simulink model "SpaceVectorPWM"  (R2022a)
settings: Solver=VariableStepAuto  StartTime=0.0  StopTime=0.5  RelTol=1e-5
model workspace (MAT data in the model file):
  Mindex = 0.795982752482
  Modulation = 5
libraries: simulink x13, spsIGBTDiodeLib x6, spsSeriesRLCBranchLib x3, spsDCVoltageSourceLib x2, spsAsynchronousMachineSIUnitsLib x1, spsMeanLib x1, spsRMSLib x1, spsGroundLib x1, spsThreePhaseVIMeasurementLib x1, spsVoltageMeasurementLib x1, spspowerguiLib x1
settings Model: Creator=Alperen  LastModifiedBy=Alperen
settings SolverCC: AlgebraicLoopSolver=TrustRegion
settings DebuggingCC: MaxConsecutiveZCsMsg=none  ModelReferenceExtraNoncontSigs=none
settings RTWCC: DLArmComputeVersion=19.05

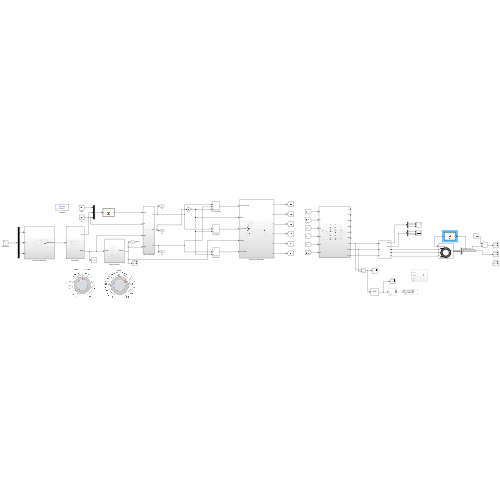
[thumbnail: Simulink's stored preview of the top-level diagram]
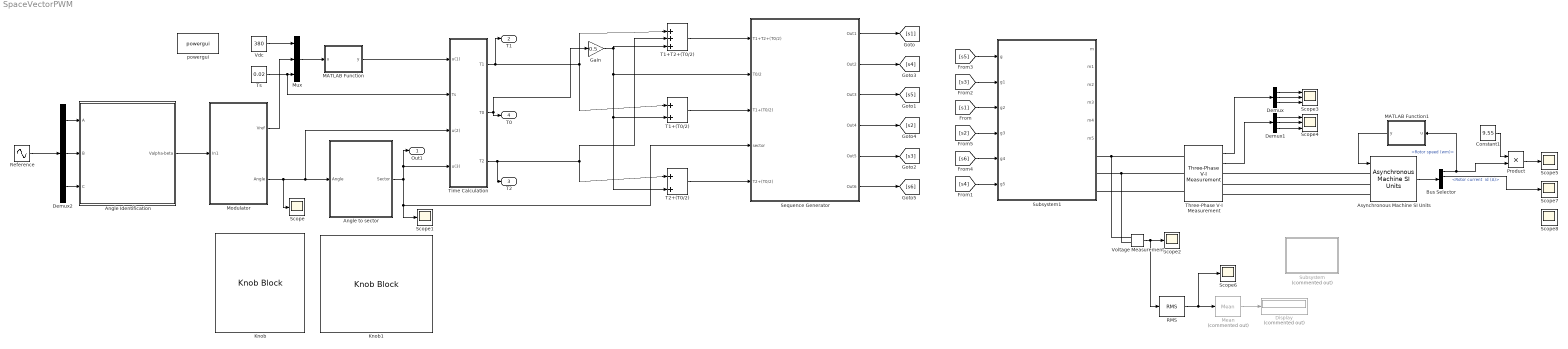
== system SpaceVectorPWM ==
  Angle Identification : Subsystem
  Angle to sector : Subsystem
  Asynchronous Machine SI Units : spsAsynchronousMachineSIUnitsLib/Asynchronous Machine SI Units  RotorType=Squirrel-cage  PresetModel="15:  5.4 HP (4KW)   400 V  50Hz 1430 RPM"  MechanicalLoad=Torque Tm  ShowDetailedParameters=on  ReferenceFrame=Rotor  Units=SI  MeasurementBus=off  NominalParameters=[4000 400 50]  VoltageRatio=1  Stator=[1.405 0.005839]  Rotor=[1.395 0.005839]  Cage1=[0.4155 0.002066]  Cage2=[0.4168 0.0003495]  Lm=0.1722  Mechanical=[0.0131 0.002985 2]  PolePairs=2  InitialConditions=[0 0 0 0 0 0 0 0]  SimulateSaturation=off  Saturation=[14.03593122, 27.81365428, 53.79336849, 72.68890987, 97.98006896, 148.6815601, 215.7428561, 302.9841135, 428.7778367 ; 230, 322, 414, 460, 506, 552, 598, 644, 690]  LoadFlowParameters=1492000  TsPowergui=0  TsBlock=-1  IterativeModel=Trapezoidal non iterative  IterativeDiscreteModel=Trapezoidal non iterative  Pmec=1.492e+006
  Bus Selector : BusSelector  OutputSignals="Mechanical.Rotor speed (wm),Rotor measurements.Rotor current  id (A),Rotor measurements.Rotor current  iq (A),Mechanical.Electromagnetic torque Te (N*m)"
  Constant1 : Constant  Value=9.55
  Demux : Demux  Outputs=3
  Demux1 : Demux  Outputs=3
  Demux2 : Demux  Outputs=3
  Display : Display  Commented=on
  Gain : Gain  Gain=0.5
  Knob : KnobBlock  TickInterval=5
  Knob1 : KnobBlock  ScaleMax=1.15  TickInterval=0.05
  MATLAB Function : MATLAB Function  TreatAsAtomicUnit=on
  MATLAB Function1 : MATLAB Function  TreatAsAtomicUnit=on
  Mean : spsMeanLib/Mean  Commented=on  Freq=50  Vinit=0  Ts=0
  Modulator : Subsystem
  Mux : Mux  Inputs=3
  Product : Product
  RMS : spsRMSLib/RMS  TrueRMS=on  Freq=50  RMSInit=390  Ts=0
  Reference : Sin  Amplitude=230  Frequency=49.62226359049479  Phase=[0 -2*pi/3 -4*pi/3]  SampleTime=0
  Scope{,1..2,5..8} (7 alike) : Scope
  Scope3 : Scope  NumInputPorts=3
  Scope4 : Scope  NumInputPorts=3
  Sequence Generator : Subsystem
  Subsystem : Subsystem  Commented=on
  Subsystem1 : Subsystem
  T1+(T0/2) : Sum  Inputs=|++
  T1+T2+(T0/2) : Sum  Inputs=|+++
  T2+(T0/2) : Sum  Inputs=|++
  Three-Phase V-I Measurement : spsThreePhaseVIMeasurementLib/Three-Phase V-I Measurement  VoltageMeasurement=phase-to-phase  SetLabelV=off  LabelV=Vabc  Vpu=off  VpuLL=off  CurrentMeasurement=yes  SetLabelI=off  LabelI=Iabc  Ipu=off  Pbase=100e6  Vbase=500e3  OutputType=Complex  PhasorSimulation=off  PSBequivalent=0
  Time Calculation : Subsystem
  Ts : Constant  Value=0.02
  Vdc : Constant  Value=380
  Voltage Measurement : spsVoltageMeasurementLib/Voltage Measurement  PhasorSimulation=off  OutputType=Complex  PSBequivalent=0
  powergui : spspowerguiLib/powergui  Priority=1  SimulationMode=Discrete  SampleTime=1e-6  frequency=60  Iterations=50  frequencyindice=0  Pbase=100e6  ErrMax=1e-4  UnitsV=kV  UnitsW=MW  buscounter=0  FunctionMessages=off  echomessages=off  EnableUseOfTLC=off  CurrentSourceSwitches=off  DisableSnubberDevices=off  DisableRonSwitches=off  DisableVfSwitches=off  DisplayEquations=off  AutomaticDiscreteSolvers=off  SolverType=Tustin/Backward Euler (TBE)  Interpol=off  ExternalGateDelay=off  methode=off  Ts=100  x0status=blocks  SPID=on  SwTol=0  HookPort=off  NonlinearTolerance=1e-4  nMaxIteration=100  ContinueOnMaxIteration=off  RestoreLinks=warning  ResistiveCurrentMeasurement=off  Frange=[0:2:500]  Ylog=off  Xlog=on  ShowGrid=off  save=off  variable=ZData  structure=0  ZoomFFT=off  StartTime=0.0  cycles=1  DisplayStyle=1  fundamental=60  FreqAxis=off  MaxFrequency=1000  frequencyindicesteady=1  RmsSteady=1  display=off
  Out1 : Outport  SignalName=sector
  T1 : Outport  Port=2
  T2 : Outport  Port=3
  T0 : Outport  Port=4
  wires:
  Angle Identification/1(Valpha-beta) -> Modulator/1(In1)
  Modulator/1(Vref) -> Mux/2
  Modulator/2(Angle) -> Time Calculation/3(u(2)), Angle to sector/1(Angle), Scope/1
  Angle to sector/1(Sector) -> Out1/1, Time Calculation/4(u(3)), Sequence Generator/4(sector), Scope1/1
  Vdc/1 -> Mux/1
  Ts/1 -> Time Calculation/2(Ts), Mux/3
  Mux/1 -> MATLAB Function/1(u)
  MATLAB Function/1(y) -> Time Calculation/1(u(1))
  Time Calculation/1(T1) -> T1/1, T1+(T0/2)/1, T1+T2+(T0/2)/1
  Time Calculation/2(T0) -> Gain/1, T0/1
  Time Calculation/3(T2) -> T2/1, T1+T2+(T0/2)/2, T2+(T0/2)/1
  Gain/1 -> T1+T2+(T0/2)/3, T1+(T0/2)/2, T2+(T0/2)/2, Sequence Generator/2(T0/2)
  Three-Phase V-I Measurement/2 -> Demux1/1
  Demux1/3 -> Scope4/3
  Demux1/1 -> Scope4/1
  Demux1/2 -> Scope4/2
  [s3] -> Subsystem1/2(g1)
  Demux/1 -> Scope3/1
  [s5] -> Subsystem1/1(g)
  Demux/2 -> Scope3/2
  [s6] -> Subsystem1/5(g4)
  [s2] -> Subsystem1/4(g3)
  [s1] -> Subsystem1/3(g2)
  [s4] -> Subsystem1/6(g5)
  Demux/3 -> Scope3/3
  T1+T2+(T0/2)/1 -> Sequence Generator/1(T1+T2+(T0/2))
  T1+(T0/2)/1 -> Sequence Generator/3(T1+(T0/2))
  T2+(T0/2)/1 -> Sequence Generator/5(T2+(T0/2))
  Sequence Generator/1(Out1) -> [s1]
  Sequence Generator/2(Out2) -> [s4]
  Sequence Generator/3(Out3) -> [s5]
  Sequence Generator/4(Out4) -> [s2]
  Sequence Generator/5(Out5) -> [s3]
  Sequence Generator/6(Out6) -> [s6]
  Reference/1 -> Demux2/1
  Demux2/3 -> Angle Identification/3(C)
  Demux2/2 -> Angle Identification/2(B)
  Demux2/1 -> Angle Identification/1(A)
  RMS/1 -> Scope6/1, Mean/1
  Voltage Measurement/1 -> RMS/1, Scope2/1
  Mean/1 -> Display/1
  Three-Phase V-I Measurement/1 -> Demux/1
  Asynchronous Machine SI Units/1 -> Bus Selector/1
  Constant1/1 -> Product/1
  Bus Selector/1 -> MATLAB Function1/1(u), Product/2  "<Rotor speed (wm)>"
  Bus Selector/2 -> Scope7/1  "<Rotor current  id (A)>"
  Product/1 -> Scope5/1
  MATLAB Function1/1(y) -> Asynchronous Machine SI Units/1
  connections:
  Three-Phase V-I Measurement/LConn3 -- Subsystem1/RConn3
  Three-Phase V-I Measurement/LConn2 -- Voltage Measurement/LConn2 -- Subsystem1/RConn2
  Three-Phase V-I Measurement/LConn1 -- Voltage Measurement/LConn1 -- Subsystem1/RConn1
  Asynchronous Machine SI Units/LConn3 -- Three-Phase V-I Measurement/RConn3
  Asynchronous Machine SI Units/LConn2 -- Three-Phase V-I Measurement/RConn2
  Asynchronous Machine SI Units/LConn1 -- Three-Phase V-I Measurement/RConn1

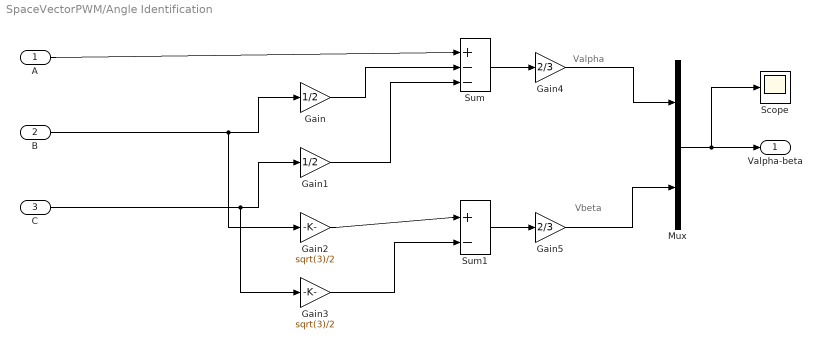
== system SpaceVectorPWM/Angle Identification ==
  note: Valpha
  note: Vbeta
  A : Inport
  B : Inport  Port=2
  C : Inport  Port=3
  Gain : Gain  Gain=1/2
  Gain1 : Gain  Gain=1/2
  Gain2 : Gain  Gain=sqrt(3)/2
  Gain3 : Gain  Gain=sqrt(3)/2
  Gain4 : Gain  Gain=2/3
  Gain5 : Gain  Gain=2/3
  Mux : Mux  Inputs=2
  Scope : Scope
  Sum : Sum  Inputs=|+--
  Sum1 : Sum  Inputs=|+-
  Valpha-beta : Outport
  wires:
  A/1 -> Sum/1
  C/1 -> Gain3/1, Gain1/1
  Sum/1 -> Gain4/1
  Gain/1 -> Sum/2
  Gain1/1 -> Sum/3
  B/1 -> Gain2/1, Gain/1
  Gain4/1 -> Mux/1
  Gain2/1 -> Sum1/1
  Gain3/1 -> Sum1/2
  Sum1/1 -> Gain5/1
  Gain5/1 -> Mux/2
  Mux/1 -> Scope/1, Valpha-beta/1

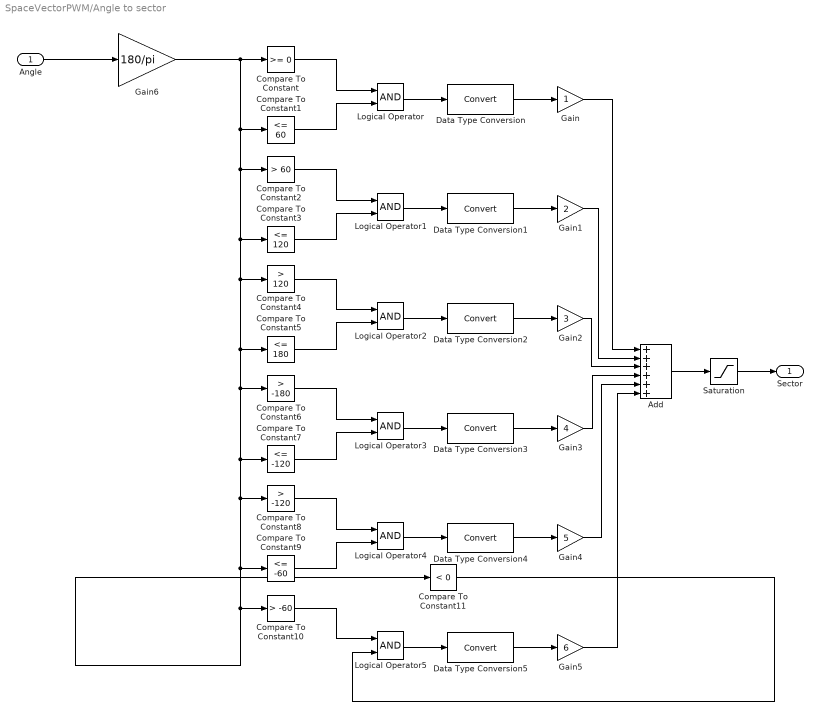
== system SpaceVectorPWM/Angle to sector ==
  Angle : Inport
  Add : Sum  Inputs=++++++
  Compare To Constant : simulink/Logic and Bit Operations/Compare To Constant  relop=>=  const=0  OutDataTypeStr=boolean
  Compare To Constant1 : simulink/Logic and Bit Operations/Compare To Constant  relop=<=  const=60  OutDataTypeStr=boolean
  Compare To Constant10 : simulink/Logic and Bit Operations/Compare To Constant  relop=>  const=-60  OutDataTypeStr=boolean
  Compare To Constant11 : simulink/Logic and Bit Operations/Compare To Constant  relop=<  const=0  OutDataTypeStr=boolean
  Compare To Constant2 : simulink/Logic and Bit Operations/Compare To Constant  relop=>  const=60  OutDataTypeStr=boolean
  Compare To Constant3 : simulink/Logic and Bit Operations/Compare To Constant  relop=<=  const=120  OutDataTypeStr=boolean
  Compare To Constant4 : simulink/Logic and Bit Operations/Compare To Constant  relop=>  const=120  OutDataTypeStr=boolean
  Compare To Constant5 : simulink/Logic and Bit Operations/Compare To Constant  relop=<=  const=180  OutDataTypeStr=boolean
  Compare To Constant6 : simulink/Logic and Bit Operations/Compare To Constant  relop=>  const=-180  OutDataTypeStr=boolean
  Compare To Constant7 : simulink/Logic and Bit Operations/Compare To Constant  relop=<=  const=-120  OutDataTypeStr=boolean
  Compare To Constant8 : simulink/Logic and Bit Operations/Compare To Constant  relop=>  const=-120  OutDataTypeStr=boolean
  Compare To Constant9 : simulink/Logic and Bit Operations/Compare To Constant  relop=<=  const=-60  OutDataTypeStr=boolean
  Data Type Conversion{,1..5} (6 alike) : DataTypeConversion  SaturateOnIntegerOverflow=off  RndMeth=Floor
  Gain : Gain
  Gain1 : Gain  Gain=2
  Gain2 : Gain  Gain=3
  Gain3 : Gain  Gain=4
  Gain4 : Gain  Gain=5
  Gain5 : Gain  Gain=6
  Gain6 : Gain  Gain=180/pi
  Logical Operator{,1..5} (6 alike) : Logic  AllPortsSameDT=off  OutDataTypeStr=boolean
  Saturation : Saturate  UpperLimit=6  LowerLimit=1
  Sector : Outport
  wires:
  Compare To Constant9/1 -> Logical Operator4/2
  Compare To Constant11/1 -> Logical Operator5/2
  Logical Operator5/1 -> Data Type Conversion5/1
  Compare To Constant2/1 -> Logical Operator1/1
  Angle/1 -> Gain6/1
  Compare To Constant3/1 -> Logical Operator1/2
  Gain6/1 -> Compare To Constant11/1, Compare To Constant10/1, Compare To Constant9/1, Compare To Constant8/1, Compare To Constant7/1, Compare To Constant6/1, Compare To Constant5/1, Compare To Constant4/1, Compare To Constant3/1, Compare To Constant2/1, Compare To Constant1/1, Compare To Constant/1
  Compare To Constant1/1 -> Logical Operator/2
  Gain3/1 -> Add/4
  Logical Operator/1 -> Data Type Conversion/1
  Data Type Conversion1/1 -> Gain1/1
  Logical Operator2/1 -> Data Type Conversion2/1
  Data Type Conversion2/1 -> Gain2/1
  Logical Operator4/1 -> Data Type Conversion4/1
  Compare To Constant5/1 -> Logical Operator2/2
  Data Type Conversion/1 -> Gain/1
  Compare To Constant8/1 -> Logical Operator4/1
  Data Type Conversion4/1 -> Gain4/1
  Logical Operator3/1 -> Data Type Conversion3/1
  Gain/1 -> Add/1
  Logical Operator1/1 -> Data Type Conversion1/1
  Compare To Constant6/1 -> Logical Operator3/1
  Data Type Conversion5/1 -> Gain5/1
  Compare To Constant/1 -> Logical Operator/1
  Data Type Conversion3/1 -> Gain3/1
  Compare To Constant7/1 -> Logical Operator3/2
  Gain2/1 -> Add/3
  Compare To Constant4/1 -> Logical Operator2/1
  Gain1/1 -> Add/2
  Compare To Constant10/1 -> Logical Operator5/1
  Gain4/1 -> Add/5
  Gain5/1 -> Add/6
  Add/1 -> Saturation/1
  Saturation/1 -> Sector/1

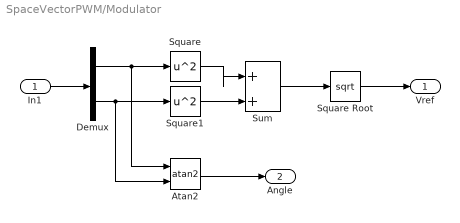
== system SpaceVectorPWM/Modulator ==
  In1 : Inport
  Atan2 : Trigonometry  Operator=atan2
  Demux : Demux  Outputs=2
  Square : Math  Operator=square
  Square Root : Sqrt
  Square1 : Math  Operator=square
  Sum : Sum  Inputs=|++
  Vref : Outport
  Angle : Outport  Port=2
  wires:
  Square Root/1 -> Vref/1
  Demux/1 -> Atan2/1, Square/1
  Demux/2 -> Atan2/2, Square1/1
  Square/1 -> Sum/1
  Sum/1 -> Square Root/1
  Square1/1 -> Sum/2
  Atan2/1 -> Angle/1
  In1/1 -> Demux/1

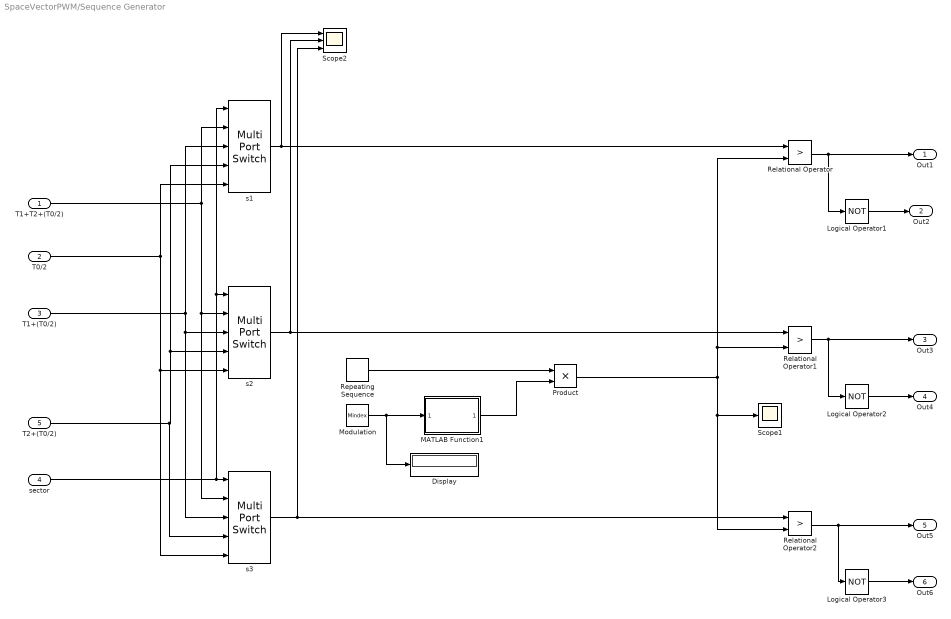
== system SpaceVectorPWM/Sequence Generator ==
  T1+T2+(T0/2) : Inport
  T0/2 : Inport  Port=2
  T1+(T0/2) : Inport  Port=3
  sector : Inport  Port=4
  T2+(T0/2) : Inport  Port=5
  Display : Display
  Logical Operator1 : Logic  Operator=NOT  AllPortsSameDT=off  OutDataTypeStr=boolean
  Logical Operator2 : Logic  Operator=NOT  AllPortsSameDT=off  OutDataTypeStr=boolean
  Logical Operator3 : Logic  Operator=NOT  AllPortsSameDT=off  OutDataTypeStr=boolean
  MATLAB Function1 : MATLAB Function  TreatAsAtomicUnit=on
  Modulation : Constant  Value=Mindex
  Product : Product
  Relational Operator : RelationalOperator  Operator=>  OutDataTypeStr=boolean  RndMeth=Simplest  InputSameDT=off
  Relational Operator1 : RelationalOperator  Operator=>  OutDataTypeStr=boolean  RndMeth=Simplest  InputSameDT=off
  Relational Operator2 : RelationalOperator  Operator=>  OutDataTypeStr=boolean  RndMeth=Simplest  InputSameDT=off
  Repeating Sequence : simulink/Sources/Repeating Sequence  rep_seq_t=[0 1e-3/4 1e-3/2 (1e-3)*3/4 1e-3]  rep_seq_y=[0,1,0,-1,0]
  Scope1 : Scope
  Scope2 : Scope  NumInputPorts=3
  s1 : MultiPortSwitch  DataPortOrder=Specify indices  Inputs=4  DataPortIndices={[1,6],2,5,[3,4]}  SaturateOnIntegerOverflow=off  InputSameDT=off
  s2 : MultiPortSwitch  DataPortOrder=Specify indices  Inputs=4  DataPortIndices={[2,3],4,1,[5,6]}  SaturateOnIntegerOverflow=off  InputSameDT=off
  s3 : MultiPortSwitch  DataPortOrder=Specify indices  Inputs=4  DataPortIndices={[4,5],6,3,[1,2]}  SaturateOnIntegerOverflow=off  InputSameDT=off
  Out1 : Outport
  Out2 : Outport  Port=2
  Out3 : Outport  Port=3
  Out4 : Outport  Port=4
  Out5 : Outport  Port=5
  Out6 : Outport  Port=6
  wires:
  T0/2/1 -> s1/5, s3/5, s2/5
  s3/1 -> Scope2/3, Relational Operator2/1
  Relational Operator1/1 -> Out3/1, Logical Operator2/1
  T1+(T0/2)/1 -> s3/3, s2/3, s1/3
  s1/1 -> Scope2/1, Relational Operator/1
  sector/1 -> s1/1, s2/1, s3/1
  s2/1 -> Scope2/2, Relational Operator1/1
  T1+T2+(T0/2)/1 -> s1/2, s3/2, s2/2
  Relational Operator/1 -> Out1/1, Logical Operator1/1
  Logical Operator3/1 -> Out6/1
  T2+(T0/2)/1 -> s3/4, s2/4, s1/4
  Relational Operator2/1 -> Out5/1, Logical Operator3/1
  Logical Operator1/1 -> Out2/1
  Logical Operator2/1 -> Out4/1
  Product/1 -> Relational Operator/2, Relational Operator1/2, Scope1/1, Relational Operator2/2
  Repeating Sequence/1 -> Product/1
  Modulation/1 -> Display/1, MATLAB Function1/1(Mindex)
  MATLAB Function1/1(Modulation) -> Product/2

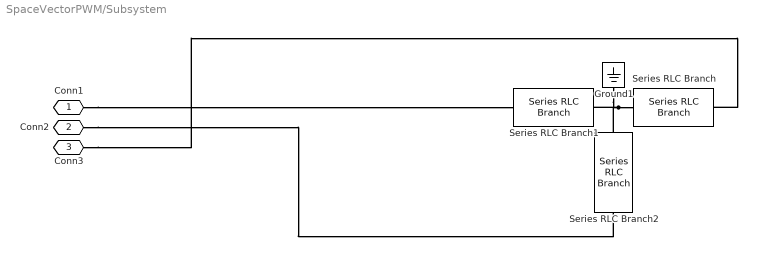
== system SpaceVectorPWM/Subsystem ==
  Ground1 : spsGroundLib/Ground  LConnTagsString=a
  Series RLC Branch : spsSeriesRLCBranchLib/Series RLC Branch  LConnTagsString=__new0  RConnTagsString=__new0  BranchType=RL  Resistance=0.3  Inductance=1e-3  SetiL0=off  InitialCurrent=0  Capacitance=0  Setx0=off  InitialVoltage=0  Measurements=None
  Series RLC Branch1 : spsSeriesRLCBranchLib/Series RLC Branch  LConnTagsString=__new0  RConnTagsString=__new0  BranchType=RL  Resistance=0.3  Inductance=1e-3  SetiL0=off  InitialCurrent=0  Capacitance=0  Setx0=off  InitialVoltage=0  Measurements=None
  Series RLC Branch2 : spsSeriesRLCBranchLib/Series RLC Branch  LConnTagsString=__new0  RConnTagsString=__new0  BranchType=RL  Resistance=0.3  Inductance=1e-3  SetiL0=off  InitialCurrent=0  Capacitance=0  Setx0=off  InitialVoltage=0  Measurements=None
  Conn1 : PMIOPort  Side=Left
  Conn2 : PMIOPort  Port=2  Side=Left
  Conn3 : PMIOPort  Port=3  Side=Left
  connections:
  Series RLC Branch/RConn1 -- Series RLC Branch2/RConn1 -- Series RLC Branch1/RConn1 -- Ground1/LConn1
  Conn3/RConn1 -- Series RLC Branch/LConn1
  Conn1/RConn1 -- Series RLC Branch1/LConn1
  Conn2/RConn1 -- Series RLC Branch2/LConn1

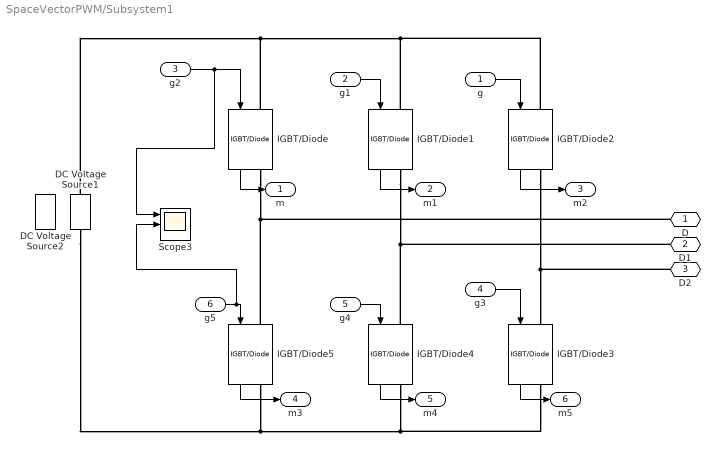
== system SpaceVectorPWM/Subsystem1 ==
  g : Inport
  g1 : Inport  Port=2
  g2 : Inport  Port=3
  g3 : Inport  Port=4
  g4 : Inport  Port=5
  g5 : Inport  Port=6
  DC Voltage Source1 : spsDCVoltageSourceLib/DC Voltage Source  Amplitude=850  Measurements=Voltage
  DC Voltage Source2 : spsDCVoltageSourceLib/DC Voltage Source  Amplitude=400  Measurements=None
  IGBT/Diode{,1..5} (6 alike) : spsIGBTDiodeLib/IGBT//Diode  Ron=1e-5  Rs=1e7  Cs=inf  Measurements=on
  Scope3 : Scope  NumInputPorts=3
  D : PMIOPort  Side=Right
  D1 : PMIOPort  Port=2  Side=Right
  D2 : PMIOPort  Port=3  Side=Right
  m : Outport
  m1 : Outport  Port=2
  m2 : Outport  Port=3
  m3 : Outport  Port=4
  m4 : Outport  Port=5
  m5 : Outport  Port=6
  wires:
  IGBT/Diode5/1 -> m3/1
  IGBT/Diode2/1 -> m2/1
  g2/1 -> Scope3/1, IGBT/Diode/1
  g1/1 -> IGBT/Diode1/1
  g/1 -> IGBT/Diode2/1
  g3/1 -> IGBT/Diode3/1
  g4/1 -> IGBT/Diode4/1
  g5/1 -> Scope3/2, IGBT/Diode5/1
  IGBT/Diode/1 -> m/1
  IGBT/Diode3/1 -> m5/1
  IGBT/Diode4/1 -> m4/1
  IGBT/Diode1/1 -> m1/1
  connections:
  IGBT/Diode5/RConn1 -- DC Voltage Source1/LConn1 -- IGBT/Diode4/RConn1 -- IGBT/Diode3/RConn1
  D2/RConn1 -- IGBT/Diode3/LConn1 -- IGBT/Diode2/RConn1
  D1/RConn1 -- IGBT/Diode4/LConn1 -- IGBT/Diode1/RConn1
  D/RConn1 -- IGBT/Diode5/LConn1 -- IGBT/Diode/RConn1
  IGBT/Diode/LConn1 -- DC Voltage Source1/RConn1 -- IGBT/Diode2/LConn1 -- IGBT/Diode1/LConn1

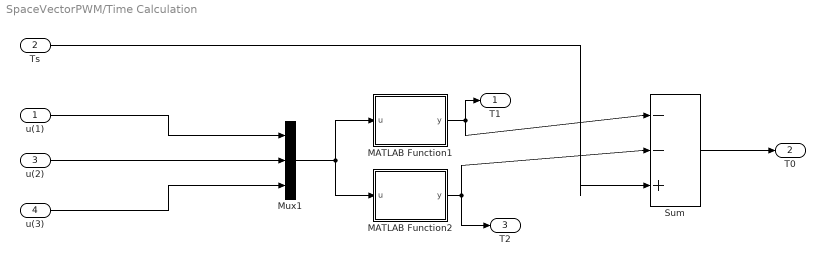
== system SpaceVectorPWM/Time Calculation ==
  u(1) : Inport
  Ts : Inport  Port=2
  u(2) : Inport  Port=3
  u(3) : Inport  Port=4
  MATLAB Function1 : MATLAB Function  TreatAsAtomicUnit=on
  MATLAB Function2 : MATLAB Function  TreatAsAtomicUnit=on
  Mux1 : Mux  Inputs=3
  Sum : Sum  Inputs=|--+
  T1 : Outport
  T0 : Outport  Port=2
  T2 : Outport  Port=3
  wires:
  MATLAB Function2/1(y) -> T2/1, Sum/2
  Sum/1 -> T0/1
  Mux1/1 -> MATLAB Function2/1(u), MATLAB Function1/1(u)
  u(2)/1 -> Mux1/2
  MATLAB Function1/1(y) -> T1/1, Sum/1
  Ts/1 -> Sum/3
  u(3)/1 -> Mux1/3
  u(1)/1 -> Mux1/1

== matlab function SpaceVectorPWM/MATLAB Function ==
  data: u input; y output
function y = fcn(u)
y=sqrt(3)*u(3)*u(2)/u(1);

== matlab function SpaceVectorPWM/Time Calculation/MATLAB Function2 ==
  data: u input; y output
function y = fcn(u)

y=u(1)*sin(-(u(3)-1)*pi/3+u(2));

== matlab function SpaceVectorPWM/Sequence Generator/MATLAB Function1 ==
  data: Mindex input; Modulation output
function Modulation  = fcn(Mindex)

Modulation = 0.0205/Mindex;

== matlab function SpaceVectorPWM/MATLAB Function1 ==
  data: u input; y output
function y = fcn(u)

y = 1.03e-3*u^2;

== matlab function SpaceVectorPWM/Time Calculation/MATLAB Function1 ==
  data: u input; y output
function y = fcn(u)

y=u(1)*sin(u(3)*pi/3-u(2));
